simulink model "Battery_Model"  (R2019b)
settings: configuration reference "BMS_Sw_CodeGenConfig" (kept outside this file)
undefined symbols (not defined in the file): Battery, TempInit, ts
libraries: fl_lib x2765, nesl_utility x1565, ee_lib x384, simulink x384, BatteryPack_lib x3
(part 2 of 33)

== system Battery_Model/Battery_Pack/Battery_Pack_7Modules/Cell_3p1 ==
  BalCmd : Inport
  AmTmp : Inport  Port=2
  CellMonitoringUnit_1 : Subsystem
  CellMonitoringUnit_2 : Subsystem
  CellMonitoringUnit_3 : Subsystem
  Cell_Module_1 : Subsystem
  Cell_Module_2 : Subsystem
  Cell_Module_3 : Subsystem
  Data Type Conversion2 : DataTypeConversion  OutDataTypeStr=double
  Data Type Conversion3 : DataTypeConversion  OutDataTypeStr=single
  Data Type Conversion4 : DataTypeConversion  OutDataTypeStr=single
  Data Type Conversion5 : DataTypeConversion  OutDataTypeStr=single
  Vector Concatenate : Concatenate  NumInputs=3
  Vector Concatenate1 : Concatenate  NumInputs=3
  Cell+ : PMIOPort  Side=Right
  Cell- : PMIOPort  Port=2  Side=Right
  Cell_Voltages : Outport  VectorParamsAs1DForOutWhenUnconnected=off
  Cell_Temperatures : Outport  Port=2  VectorParamsAs1DForOutWhenUnconnected=off
  wires:
  Data Type Conversion4/1 -> [Module01_Volts]
  CellMonitoringUnit_1/1(CellVoltages) -> Data Type Conversion4/1
  Data Type Conversion2/1 -> CellMonitoringUnit_3/1(BalCmd), CellMonitoringUnit_2/1(BalCmd), CellMonitoringUnit_1/1(BalCmd)
  [Module01_Volts] -> Vector Concatenate/1  "Module01_Volts"
  Data Type Conversion5/1 -> [Module03_Volts]
  AmTmp/1 -> Cell_Module_3/1(AmbientTemp), Cell_Module_2/1(AmbientTemp), Cell_Module_1/1(AmbientTemp)
  CellMonitoringUnit_2/1(CellVoltages) -> Data Type Conversion3/1
  Data Type Conversion3/1 -> [Module02_Volts]
  Cell_Module_1/1(CellTemp) -> [Module01_Temps]
  Cell_Module_2/1(CellTemp) -> [Module02_Temps]
  BalCmd/1 -> Data Type Conversion2/1
  CellMonitoringUnit_3/1(CellVoltages) -> Data Type Conversion5/1
  [Module03_Volts] -> Vector Concatenate/3  "Module03_Volts"
  Vector Concatenate/1 -> Cell_Voltages/1
  [Module02_Volts] -> Vector Concatenate/2  "Module02_Volts"
  Cell_Module_3/1(CellTemp) -> [Module03_Temps]
  [Module03_Temps] -> Vector Concatenate1/3
  [Module01_Temps] -> Vector Concatenate1/1
  [Module02_Temps] -> Vector Concatenate1/2
  Vector Concatenate1/1 -> Cell_Temperatures/1
  connections:
  CellMonitoringUnit_1/LConn9 -- Cell_Module_1/RConn9
  Cell_Module_3/RConn6 -- CellMonitoringUnit_3/LConn6
  Cell_Module_2/RConn11 -- CellMonitoringUnit_2/LConn11
  Cell_Module_3/RConn9 -- CellMonitoringUnit_3/LConn9
  Cell_Module_2/RConn5 -- CellMonitoringUnit_2/LConn5
  CellMonitoringUnit_1/LConn13 -- Cell_Module_1/RConn13
  Cell_Module_2/RConn6 -- CellMonitoringUnit_2/LConn6
  Cell_Module_1/RConn17 -- Cell-/RConn1 -- CellMonitoringUnit_2/LConn17 -- CellMonitoringUnit_3/LConn17 -- Cell_Module_3/RConn17 -- Cell_Module_2/RConn17 -- CellMonitoringUnit_1/LConn17
  CellMonitoringUnit_1/LConn8 -- Cell_Module_1/RConn8
  Cell_Module_2/RConn13 -- CellMonitoringUnit_2/LConn13
  Cell_Module_2/RConn8 -- CellMonitoringUnit_2/LConn8
  CellMonitoringUnit_1/LConn1 -- Cell_Module_3/RConn1 -- CellMonitoringUnit_3/LConn1 -- Cell_Module_2/RConn1 -- CellMonitoringUnit_2/LConn1 -- Cell_Module_1/RConn1 -- Cell+/RConn1
  CellMonitoringUnit_1/LConn7 -- Cell_Module_1/RConn7
  Cell_Module_2/RConn10 -- CellMonitoringUnit_2/LConn10
  Cell_Module_3/RConn3 -- CellMonitoringUnit_3/LConn3
  Cell_Module_2/RConn14 -- CellMonitoringUnit_2/LConn14
  Cell_Module_2/RConn16 -- CellMonitoringUnit_2/LConn16
  Cell_Module_2/RConn12 -- CellMonitoringUnit_2/LConn12
  Cell_Module_2/RConn2 -- CellMonitoringUnit_2/LConn2
  Cell_Module_3/RConn4 -- CellMonitoringUnit_3/LConn4
  Cell_Module_3/RConn2 -- CellMonitoringUnit_3/LConn2
  Cell_Module_3/RConn8 -- CellMonitoringUnit_3/LConn8
  CellMonitoringUnit_1/LConn11 -- Cell_Module_1/RConn11
  Cell_Module_2/RConn9 -- CellMonitoringUnit_2/LConn9
  Cell_Module_3/RConn12 -- CellMonitoringUnit_3/LConn12
  CellMonitoringUnit_1/LConn3 -- Cell_Module_1/RConn3
  CellMonitoringUnit_1/LConn15 -- Cell_Module_1/RConn15
  Cell_Module_3/RConn7 -- CellMonitoringUnit_3/LConn7
  CellMonitoringUnit_1/LConn5 -- Cell_Module_1/RConn5
  Cell_Module_3/RConn15 -- CellMonitoringUnit_3/LConn15
  CellMonitoringUnit_1/LConn12 -- Cell_Module_1/RConn12
  CellMonitoringUnit_1/LConn10 -- Cell_Module_1/RConn10
  Cell_Module_2/RConn3 -- CellMonitoringUnit_2/LConn3
  CellMonitoringUnit_1/LConn6 -- Cell_Module_1/RConn6
  Cell_Module_2/RConn4 -- CellMonitoringUnit_2/LConn4
  Cell_Module_3/RConn10 -- CellMonitoringUnit_3/LConn10
  CellMonitoringUnit_1/LConn14 -- Cell_Module_1/RConn14
  CellMonitoringUnit_1/LConn4 -- Cell_Module_1/RConn4
  Cell_Module_3/RConn16 -- CellMonitoringUnit_3/LConn16
  Cell_Module_3/RConn11 -- CellMonitoringUnit_3/LConn11
  Cell_Module_3/RConn13 -- CellMonitoringUnit_3/LConn13
  Cell_Module_3/RConn14 -- CellMonitoringUnit_3/LConn14
  Cell_Module_3/RConn5 -- CellMonitoringUnit_3/LConn5
  Cell_Module_2/RConn15 -- CellMonitoringUnit_2/LConn15
  Cell_Module_2/RConn7 -- CellMonitoringUnit_2/LConn7
  CellMonitoringUnit_1/LConn2 -- Cell_Module_1/RConn2
  CellMonitoringUnit_1/LConn16 -- Cell_Module_1/RConn16

== system Battery_Model/Battery_Pack/Battery_Pack_1Module/Cell_3p/CellMonitoringUnit_1 ==
  BalCmd : Inport
  D{1..4,7..9,13..16} (11 alike) : fl_lib/Electrical/Electrical Elements/Diode  Vf=0.6 V  Ron=0.3 Ohm  Goff=1e-8 1/Ohm  i_specify=off  i_priority=High  i=0 A  i_nominal_specify=off  i_nominal_unit=A  i_nominal_value=1  v_specify=off  v_priority=None  v=0 V  v_nominal_specify=off  v_nominal_unit=V  v_nominal_value=1
      settings: LogSimulationData=on
  D{5..6,10..12} (5 alike) : fl_lib/Electrical/Electrical Elements/Diode  Vf=0.6 V  Ron=0.3 Ohm  Goff=1e-8 1/Ohm  i_specify=off  i_priority=None  i=0 A  i_nominal_specify=off  i_nominal_unit=A  i_nominal_value=1  v_specify=off  v_priority=None  v=0 V  v_nominal_specify=off  v_nominal_unit=V  v_nominal_value=1
      settings: LogSimulationData=on
  Data Type Conversion{,1..15} (16 alike) : DataTypeConversion  OutDataTypeStr=single
  PS-Simulink Converter{1..12,14..17} (16 alike) : nesl_utility/PS-Simulink Converter  PhysicalDomain=network_engine_domain  SubClassName=ps_output  LeftPortType=input  RightPortType=output  PseudoPeriodic=off  Frequencies=[]  Unit=V  AffineConversion=off
  R{1..16} (16 alike) : fl_lib/Electrical/Electrical Elements/Resistor  R=Battery.R_bleed Ohm  i_specify=off  i_priority=None  i=0 A  i_nominal_specify=off  i_nominal_unit=A  i_nominal_value=1  v_specify=off  v_priority=None  v=0 V  v_nominal_specify=off  v_nominal_unit=V  v_nominal_value=1
      R1 settings: LogSimulationData=on
  Selector : Selector  IndexOptions=Index vector (dialog)  Indices=1  OutputSizes=1
  Selector1 : Selector  IndexOptions=Index vector (dialog)  Indices=2  OutputSizes=1
  Selector10 : Selector  IndexOptions=Index vector (dialog)  Indices=6  OutputSizes=1
  Selector{3,8,11,15} (4 alike) : Selector  IndexOptions=Index vector (dialog)  Indices=4  OutputSizes=1
  Selector12 : Selector  IndexOptions=Index vector (dialog)  Indices=6  OutputSizes=1
  Selector13 : Selector  IndexOptions=Index vector (dialog)  Indices=2  OutputSizes=1
  Selector14 : Selector  IndexOptions=Index vector (dialog)  Indices=3  OutputSizes=1
  Selector2 : Selector  IndexOptions=Index vector (dialog)  Indices=3  OutputSizes=1
  Selector4 : Selector  IndexOptions=Index vector (dialog)  Indices=5  OutputSizes=1
  Selector5 : Selector  IndexOptions=Index vector (dialog)  Indices=6  OutputSizes=1
  Selector6 : Selector  IndexOptions=Index vector (dialog)  Indices=2  OutputSizes=1
  Selector7 : Selector  IndexOptions=Index vector (dialog)  Indices=3  OutputSizes=1
  Selector9 : Selector  IndexOptions=Index vector (dialog)  Indices=5  OutputSizes=1
  Simulink-PS Converter{1..12,14..17} (16 alike) : nesl_utility/Simulink-PS Converter  PhysicalDomain=network_engine_domain  SubClassName=ps_input  LeftPortType=input  RightPortType=output  PseudoPeriodic=off  Frequencies=[]  NoiseDistribution=none  NoiseParameters=[]  Unit=1  AffineConversion=off  FilteringAndDerivatives=zero  SimscapeFilterOrder=1  InputFilterTimeConstant=0.001  UdotUserProvided=1
  Switch{,1..15} (16 alike) : fl_lib/Electrical/Electrical Elements/Switch  R_closed=0.01 Ohm  G_open=1e-8 1/Ohm  Threshold=0  i_specify=off  i_priority=None  i=0 A  i_nominal_specify=off  i_nominal_unit=A  i_nominal_value=1  v_specify=off  v_priority=None  v=0 V  v_nominal_specify=off  v_nominal_unit=V  v_nominal_value=1
      settings: SourceProductName=Simscape
  Vector Concatenate : Concatenate  NumInputs=16
  Voltage Sensor{1..12,14..17} (16 alike) : fl_lib/Electrical/Electrical Sensors/Voltage Sensor
  Conn1 : PMIOPort  Side=Left
  Conn2 : PMIOPort  Port=2  Side=Left
  Conn3 : PMIOPort  Port=3  Side=Left
  Conn4 : PMIOPort  Port=4  Side=Left
  Conn5 : PMIOPort  Port=5  Side=Left
  Conn6 : PMIOPort  Port=6  Side=Left
  Conn7 : PMIOPort  Port=7  Side=Left
  Conn8 : PMIOPort  Port=8  Side=Left
  Conn9 : PMIOPort  Port=9  Side=Left
  Conn10 : PMIOPort  Port=10  Side=Left
  Conn11 : PMIOPort  Port=11  Side=Left
  Conn12 : PMIOPort  Port=12  Side=Left
  Conn13 : PMIOPort  Port=13  Side=Left
  Conn14 : PMIOPort  Port=14  Side=Left
  Conn15 : PMIOPort  Port=15  Side=Left
  Conn16 : PMIOPort  Port=16  Side=Left
  Conn17 : PMIOPort  Port=17  Side=Left
  CellVoltages : Outport  VectorParamsAs1DForOutWhenUnconnected=off
  wires:
  BalCmd/1 -> Selector/1, Selector1/1, Selector11/1, Selector15/1, Selector14/1, Selector13/1, Selector12/1, Selector10/1, Selector9/1, Selector8/1, Selector7/1, Selector6/1, Selector5/1, Selector4/1, Selector3/1, Selector2/1
  PS-Simulink Converter8/1 -> Data Type Conversion8/1  "Cell9_Volt"
  Selector5/1 -> Simulink-PS Converter6/1
  PS-Simulink Converter10/1 -> Data Type Conversion9/1  "Cell10_Volt"
  Selector9/1 -> Simulink-PS Converter10/1
  Data Type Conversion3/1 -> Vector Concatenate/4  "Cell4_Volt"
  Data Type Conversion12/1 -> Vector Concatenate/12  "Cell12_Volt"
  Selector6/1 -> Simulink-PS Converter7/1
  PS-Simulink Converter12/1 -> Data Type Conversion11/1  "Cell16_Volt"
  Data Type Conversion8/1 -> Vector Concatenate/9  "Cell9_Volt"
  Selector2/1 -> Simulink-PS Converter4/1
  Data Type Conversion/1 -> Vector Concatenate/1  "Cell1_Volt"
  Selector8/1 -> Simulink-PS Converter8/1
  Data Type Conversion15/1 -> Vector Concatenate/15  "Cell15_Volt"
  Data Type Conversion11/1 -> Vector Concatenate/16  "Cell16_Volt"
  Selector10/1 -> Simulink-PS Converter11/1
  PS-Simulink Converter15/1 -> Data Type Conversion14/1  "Cell14_Volt"
  Data Type Conversion4/1 -> Vector Concatenate/5  "Cell5_Volt"
  PS-Simulink Converter9/1 -> Data Type Conversion6/1  "Cell7_Volt"
  PS-Simulink Converter11/1 -> Data Type Conversion10/1  "Cell11_Volt"
  Data Type Conversion2/1 -> Vector Concatenate/3  "Cell3_Volt"
  Data Type Conversion7/1 -> Vector Concatenate/8  "Cell8_Volt"
  PS-Simulink Converter7/1 -> Data Type Conversion7/1  "Cell8_Volt"
  Selector7/1 -> Simulink-PS Converter9/1
  Selector12/1 -> Simulink-PS Converter14/1
  PS-Simulink Converter14/1 -> Data Type Conversion12/1  "Cell12_Volt"
  Selector15/1 -> Simulink-PS Converter16/1
  Selector14/1 -> Simulink-PS Converter17/1
  PS-Simulink Converter17/1 -> Data Type Conversion13/1  "Cell13_Volt"
  Data Type Conversion13/1 -> Vector Concatenate/13  "Cell13_Volt"
  PS-Simulink Converter16/1 -> Data Type Conversion15/1  "Cell15_Volt"
  Selector13/1 -> Simulink-PS Converter15/1
  Data Type Conversion1/1 -> Vector Concatenate/2  "Cell2_Volt"
  Data Type Conversion9/1 -> Vector Concatenate/10  "Cell10_Volt"
  PS-Simulink Converter6/1 -> Data Type Conversion5/1  "Cell6_Volt"
  PS-Simulink Converter4/1 -> Data Type Conversion1/1  "Cell2_Volt"
  Selector11/1 -> Simulink-PS Converter12/1
  Data Type Conversion14/1 -> Vector Concatenate/14  "Cell14_Volt"
  Vector Concatenate/1 -> CellVoltages/1
  Selector4/1 -> Simulink-PS Converter5/1
  Selector1/1 -> Simulink-PS Converter1/1
  PS-Simulink Converter2/1 -> Data Type Conversion/1  "Cell1_Volt"
  Selector3/1 -> Simulink-PS Converter2/1
  PS-Simulink Converter1/1 -> Data Type Conversion2/1  "Cell3_Volt"
  Selector/1 -> Simulink-PS Converter3/1
  PS-Simulink Converter3/1 -> Data Type Conversion3/1  "Cell4_Volt"
  PS-Simulink Converter5/1 -> Data Type Conversion4/1  "Cell5_Volt"
  Data Type Conversion5/1 -> Vector Concatenate/6  "Cell6_Volt"
  Data Type Conversion6/1 -> Vector Concatenate/7  "Cell7_Volt"
  Data Type Conversion10/1 -> Vector Concatenate/11  "Cell11_Volt"
  connections:
  Voltage Sensor10/RConn1 -- PS-Simulink Converter10/LConn1
  Simulink-PS Converter16/RConn1 -- Switch15/RConn1
  Switch15/RConn2 -- Voltage Sensor12/LConn1 -- Voltage Sensor17/RConn2 -- R16/LConn1 -- Conn16/RConn1
  R5/LConn1 -- Voltage Sensor5/LConn1 -- Voltage Sensor4/RConn2 -- Switch3/RConn2 -- Conn5/RConn1
  Switch12/RConn2 -- Voltage Sensor15/LConn1 -- Voltage Sensor14/RConn2 -- R13/LConn1 -- Conn13/RConn1
  Switch9/RConn2 -- R11/LConn1 -- Voltage Sensor11/LConn1 -- Voltage Sensor10/RConn2 -- Conn11/RConn1
  Switch7/LConn1 -- D8/RConn1
  Simulink-PS Converter10/RConn1 -- Switch9/RConn1
  Switch13/LConn1 -- D13/RConn1
  Voltage Sensor4/RConn1 -- PS-Simulink Converter3/LConn1
  Switch13/RConn2 -- R14/LConn1 -- Voltage Sensor16/LConn1 -- Voltage Sensor15/RConn2 -- Conn14/RConn1
  Voltage Sensor12/RConn1 -- PS-Simulink Converter12/LConn1
  Voltage Sensor14/LConn1 -- Voltage Sensor11/RConn2 -- R12/LConn1 -- Switch10/RConn2 -- Conn12/RConn1
  Simulink-PS Converter4/RConn1 -- Switch2/RConn1
  Simulink-PS Converter7/RConn1 -- Switch6/RConn1
  R11/RConn1 -- D11/LConn1
  Voltage Sensor14/RConn1 -- PS-Simulink Converter14/LConn1
  Voltage Sensor7/RConn1 -- PS-Simulink Converter9/LConn1
  Voltage Sensor9/RConn1 -- PS-Simulink Converter8/LConn1
  Switch9/LConn1 -- D10/RConn1
  R8/RConn1 -- D8/LConn1
  R9/RConn1 -- D9/LConn1
  Voltage Sensor16/RConn1 -- PS-Simulink Converter15/LConn1
  Simulink-PS Converter6/RConn1 -- Switch5/RConn1
  Simulink-PS Converter9/RConn1 -- Switch7/RConn1
  R7/RConn1 -- D7/LConn1
  Switch8/LConn1 -- D9/RConn1
  Simulink-PS Converter8/RConn1 -- Switch8/RConn1
  R3/RConn1 -- D3/LConn1
  Switch6/LConn1 -- D7/RConn1
  Switch4/RConn2 -- Voltage Sensor6/LConn1 -- Voltage Sensor5/RConn2 -- R6/LConn1 -- Conn6/RConn1
  Voltage Sensor17/RConn1 -- PS-Simulink Converter16/LConn1
  Switch3/LConn1 -- D4/RConn1
  Switch6/RConn2 -- R8/LConn1 -- Voltage Sensor7/RConn2 -- Voltage Sensor8/LConn1 -- Conn8/RConn1
  Switch/RConn2 -- R2/LConn1 -- Voltage Sensor2/LConn1 -- Voltage Sensor1/RConn2 -- Conn2/RConn1
  Switch15/LConn1 -- D15/RConn1
  Voltage Sensor9/RConn2 -- Voltage Sensor10/LConn1 -- R10/LConn1 -- Switch8/RConn2 -- Conn10/RConn1
  Voltage Sensor7/LConn1 -- Voltage Sensor6/RConn2 -- R7/LConn1 -- Switch5/RConn2 -- Conn7/RConn1
  Switch2/RConn2 -- R4/LConn1 -- Voltage Sensor4/LConn1 -- Voltage Sensor3/RConn2 -- Conn4/RConn1
  R12/RConn1 -- D12/LConn1
  Voltage Sensor11/RConn1 -- PS-Simulink Converter11/LConn1
  Simulink-PS Converter14/RConn1 -- Switch12/RConn1
  R14/RConn1 -- D14/LConn1
  Simulink-PS Converter17/RConn1 -- Switch14/RConn1
  Switch14/RConn2 -- R15/LConn1 -- Voltage Sensor17/LConn1 -- Voltage Sensor16/RConn2 -- Conn15/RConn1
  Switch12/LConn1 -- D12/RConn1
  Simulink-PS Converter2/RConn1 -- Switch3/RConn1
  R13/RConn1 -- D13/LConn1
  Switch14/LConn1 -- D14/RConn1
  Voltage Sensor15/RConn1 -- PS-Simulink Converter17/LConn1
  Switch11/RConn2 -- Voltage Sensor12/RConn2 -- Conn17/RConn1
  R15/RConn1 -- D15/LConn1
  Simulink-PS Converter15/RConn1 -- Switch13/RConn1
  Switch5/LConn1 -- D6/RConn1
  Switch7/RConn2 -- R9/LConn1 -- Voltage Sensor9/LConn1 -- Voltage Sensor8/RConn2 -- Conn9/RConn1
  Voltage Sensor8/RConn1 -- PS-Simulink Converter7/LConn1
  R1/LConn1 -- Voltage Sensor1/LConn1 -- Conn1/RConn1
  Voltage Sensor3/LConn1 -- Voltage Sensor2/RConn2 -- R3/LConn1 -- Switch1/RConn2 -- Conn3/RConn1
  Simulink-PS Converter12/RConn1 -- Switch11/RConn1
  Simulink-PS Converter1/RConn1 -- Switch1/RConn1
  PS-Simulink Converter2/LConn1 -- Voltage Sensor1/RConn1
  R4/RConn1 -- D4/LConn1
  Switch1/LConn1 -- D2/RConn1
  R2/RConn1 -- D2/LConn1
  Simulink-PS Converter5/RConn1 -- Switch4/RConn1
  Switch2/LConn1 -- D3/RConn1
  Simulink-PS Converter3/RConn1 -- Switch/RConn1
  Switch4/LConn1 -- D5/RConn1
  Voltage Sensor2/RConn1 -- PS-Simulink Converter4/LConn1
  R1/RConn1 -- D1/LConn1
  R5/RConn1 -- D5/LConn1
  Voltage Sensor3/RConn1 -- PS-Simulink Converter1/LConn1
  Switch/LConn1 -- D1/RConn1
  R6/RConn1 -- D6/LConn1
  Voltage Sensor5/RConn1 -- PS-Simulink Converter5/LConn1
  R10/RConn1 -- D10/LConn1
  Voltage Sensor6/RConn1 -- PS-Simulink Converter6/LConn1
  Simulink-PS Converter11/RConn1 -- Switch10/RConn1
  Switch10/LConn1 -- D11/RConn1
  R16/RConn1 -- D16/LConn1
  Switch11/LConn1 -- D16/RConn1

== system Battery_Model/Battery_Pack/Battery_Pack_1Module/Cell_3p/CellMonitoringUnit_2 ==
  BalCmd : Inport
  D{1..4,7..9,13..16} (11 alike) : fl_lib/Electrical/Electrical Elements/Diode  Vf=0.6 V  Ron=0.3 Ohm  Goff=1e-8 1/Ohm  i_specify=off  i_priority=High  i=0 A  i_nominal_specify=off  i_nominal_unit=A  i_nominal_value=1  v_specify=off  v_priority=None  v=0 V  v_nominal_specify=off  v_nominal_unit=V  v_nominal_value=1
      settings: LogSimulationData=on
  D{5..6,10..12} (5 alike) : fl_lib/Electrical/Electrical Elements/Diode  Vf=0.6 V  Ron=0.3 Ohm  Goff=1e-8 1/Ohm  i_specify=off  i_priority=None  i=0 A  i_nominal_specify=off  i_nominal_unit=A  i_nominal_value=1  v_specify=off  v_priority=None  v=0 V  v_nominal_specify=off  v_nominal_unit=V  v_nominal_value=1
      settings: LogSimulationData=on
  Data Type Conversion{,1..15} (16 alike) : DataTypeConversion  OutDataTypeStr=single
  PS-Simulink Converter{1..12,14..17} (16 alike) : nesl_utility/PS-Simulink Converter  PhysicalDomain=network_engine_domain  SubClassName=ps_output  LeftPortType=input  RightPortType=output  PseudoPeriodic=off  Frequencies=[]  Unit=V  AffineConversion=off
  R{1..16} (16 alike) : fl_lib/Electrical/Electrical Elements/Resistor  R=Battery.R_bleed Ohm  i_specify=off  i_priority=None  i=0 A  i_nominal_specify=off  i_nominal_unit=A  i_nominal_value=1  v_specify=off  v_priority=None  v=0 V  v_nominal_specify=off  v_nominal_unit=V  v_nominal_value=1
      R1 settings: LogSimulationData=on
  Selector : Selector  IndexOptions=Index vector (dialog)  Indices=1  OutputSizes=1
  Selector1 : Selector  IndexOptions=Index vector (dialog)  Indices=2  OutputSizes=1
  Selector10 : Selector  IndexOptions=Index vector (dialog)  Indices=6  OutputSizes=1
  Selector{3,8,11,15} (4 alike) : Selector  IndexOptions=Index vector (dialog)  Indices=4  OutputSizes=1
  Selector12 : Selector  IndexOptions=Index vector (dialog)  Indices=6  OutputSizes=1
  Selector13 : Selector  IndexOptions=Index vector (dialog)  Indices=2  OutputSizes=1
  Selector14 : Selector  IndexOptions=Index vector (dialog)  Indices=3  OutputSizes=1
  Selector2 : Selector  IndexOptions=Index vector (dialog)  Indices=3  OutputSizes=1
  Selector4 : Selector  IndexOptions=Index vector (dialog)  Indices=5  OutputSizes=1
  Selector5 : Selector  IndexOptions=Index vector (dialog)  Indices=6  OutputSizes=1
  Selector6 : Selector  IndexOptions=Index vector (dialog)  Indices=2  OutputSizes=1
  Selector7 : Selector  IndexOptions=Index vector (dialog)  Indices=3  OutputSizes=1
  Selector9 : Selector  IndexOptions=Index vector (dialog)  Indices=5  OutputSizes=1
  Simulink-PS Converter{1..12,14..17} (16 alike) : nesl_utility/Simulink-PS Converter  PhysicalDomain=network_engine_domain  SubClassName=ps_input  LeftPortType=input  RightPortType=output  PseudoPeriodic=off  Frequencies=[]  NoiseDistribution=none  NoiseParameters=[]  Unit=1  AffineConversion=off  FilteringAndDerivatives=zero  SimscapeFilterOrder=1  InputFilterTimeConstant=0.001  UdotUserProvided=1
  Switch{,1..15} (16 alike) : fl_lib/Electrical/Electrical Elements/Switch  R_closed=0.01 Ohm  G_open=1e-8 1/Ohm  Threshold=0  i_specify=off  i_priority=None  i=0 A  i_nominal_specify=off  i_nominal_unit=A  i_nominal_value=1  v_specify=off  v_priority=None  v=0 V  v_nominal_specify=off  v_nominal_unit=V  v_nominal_value=1
      settings: SourceProductName=Simscape
  Vector Concatenate : Concatenate  NumInputs=16
  Voltage Sensor{1..12,14..17} (16 alike) : fl_lib/Electrical/Electrical Sensors/Voltage Sensor
  Conn1 : PMIOPort  Side=Left
  Conn2 : PMIOPort  Port=2  Side=Left
  Conn3 : PMIOPort  Port=3  Side=Left
  Conn4 : PMIOPort  Port=4  Side=Left
  Conn5 : PMIOPort  Port=5  Side=Left
  Conn6 : PMIOPort  Port=6  Side=Left
  Conn7 : PMIOPort  Port=7  Side=Left
  Conn8 : PMIOPort  Port=8  Side=Left
  Conn9 : PMIOPort  Port=9  Side=Left
  Conn10 : PMIOPort  Port=10  Side=Left
  Conn11 : PMIOPort  Port=11  Side=Left
  Conn12 : PMIOPort  Port=12  Side=Left
  Conn13 : PMIOPort  Port=13  Side=Left
  Conn14 : PMIOPort  Port=14  Side=Left
  Conn15 : PMIOPort  Port=15  Side=Left
  Conn16 : PMIOPort  Port=16  Side=Left
  Conn17 : PMIOPort  Port=17  Side=Left
  CellVoltages : Outport  VectorParamsAs1DForOutWhenUnconnected=off
  wires:
  BalCmd/1 -> Selector/1, Selector1/1, Selector11/1, Selector15/1, Selector14/1, Selector13/1, Selector12/1, Selector10/1, Selector9/1, Selector8/1, Selector7/1, Selector6/1, Selector5/1, Selector4/1, Selector3/1, Selector2/1
  PS-Simulink Converter8/1 -> Data Type Conversion8/1  "Cell9_Volt"
  Selector5/1 -> Simulink-PS Converter6/1
  PS-Simulink Converter10/1 -> Data Type Conversion9/1  "Cell10_Volt"
  Selector9/1 -> Simulink-PS Converter10/1
  Data Type Conversion3/1 -> Vector Concatenate/4  "Cell4_Volt"
  Data Type Conversion12/1 -> Vector Concatenate/12  "Cell12_Volt"
  Selector6/1 -> Simulink-PS Converter7/1
  PS-Simulink Converter12/1 -> Data Type Conversion11/1  "Cell16_Volt"
  Data Type Conversion8/1 -> Vector Concatenate/9  "Cell9_Volt"
  Selector2/1 -> Simulink-PS Converter4/1
  Data Type Conversion/1 -> Vector Concatenate/1  "Cell1_Volt"
  Selector8/1 -> Simulink-PS Converter8/1
  Data Type Conversion15/1 -> Vector Concatenate/15  "Cell15_Volt"
  Data Type Conversion11/1 -> Vector Concatenate/16  "Cell16_Volt"
  Selector10/1 -> Simulink-PS Converter11/1
  PS-Simulink Converter15/1 -> Data Type Conversion14/1  "Cell14_Volt"
  Data Type Conversion4/1 -> Vector Concatenate/5  "Cell5_Volt"
  PS-Simulink Converter9/1 -> Data Type Conversion6/1  "Cell7_Volt"
  PS-Simulink Converter11/1 -> Data Type Conversion10/1  "Cell11_Volt"
  Data Type Conversion2/1 -> Vector Concatenate/3  "Cell3_Volt"
  Data Type Conversion7/1 -> Vector Concatenate/8  "Cell8_Volt"
  PS-Simulink Converter7/1 -> Data Type Conversion7/1  "Cell8_Volt"
  Selector7/1 -> Simulink-PS Converter9/1
  Selector12/1 -> Simulink-PS Converter14/1
  PS-Simulink Converter14/1 -> Data Type Conversion12/1  "Cell12_Volt"
  Selector15/1 -> Simulink-PS Converter16/1
  Selector14/1 -> Simulink-PS Converter17/1
  PS-Simulink Converter17/1 -> Data Type Conversion13/1  "Cell13_Volt"
  Data Type Conversion13/1 -> Vector Concatenate/13  "Cell13_Volt"
  PS-Simulink Converter16/1 -> Data Type Conversion15/1  "Cell15_Volt"
  Selector13/1 -> Simulink-PS Converter15/1
  Data Type Conversion1/1 -> Vector Concatenate/2  "Cell2_Volt"
  Data Type Conversion9/1 -> Vector Concatenate/10  "Cell10_Volt"
  PS-Simulink Converter6/1 -> Data Type Conversion5/1  "Cell6_Volt"
  PS-Simulink Converter4/1 -> Data Type Conversion1/1  "Cell2_Volt"
  Selector11/1 -> Simulink-PS Converter12/1
  Data Type Conversion14/1 -> Vector Concatenate/14  "Cell14_Volt"
  Vector Concatenate/1 -> CellVoltages/1
  Selector4/1 -> Simulink-PS Converter5/1
  Selector1/1 -> Simulink-PS Converter1/1
  PS-Simulink Converter2/1 -> Data Type Conversion/1  "Cell1_Volt"
  Selector3/1 -> Simulink-PS Converter2/1
  PS-Simulink Converter1/1 -> Data Type Conversion2/1  "Cell3_Volt"
  Selector/1 -> Simulink-PS Converter3/1
  PS-Simulink Converter3/1 -> Data Type Conversion3/1  "Cell4_Volt"
  PS-Simulink Converter5/1 -> Data Type Conversion4/1  "Cell5_Volt"
  Data Type Conversion5/1 -> Vector Concatenate/6  "Cell6_Volt"
  Data Type Conversion6/1 -> Vector Concatenate/7  "Cell7_Volt"
  Data Type Conversion10/1 -> Vector Concatenate/11  "Cell11_Volt"
  connections:
  Voltage Sensor10/RConn1 -- PS-Simulink Converter10/LConn1
  Simulink-PS Converter16/RConn1 -- Switch15/RConn1
  Switch15/RConn2 -- Voltage Sensor12/LConn1 -- Voltage Sensor17/RConn2 -- R16/LConn1 -- Conn16/RConn1
  R5/LConn1 -- Voltage Sensor5/LConn1 -- Voltage Sensor4/RConn2 -- Switch3/RConn2 -- Conn5/RConn1
  Switch12/RConn2 -- Voltage Sensor15/LConn1 -- Voltage Sensor14/RConn2 -- R13/LConn1 -- Conn13/RConn1
  Switch9/RConn2 -- R11/LConn1 -- Voltage Sensor11/LConn1 -- Voltage Sensor10/RConn2 -- Conn11/RConn1
  Switch7/LConn1 -- D8/RConn1
  Simulink-PS Converter10/RConn1 -- Switch9/RConn1
  Switch13/LConn1 -- D13/RConn1
  Voltage Sensor4/RConn1 -- PS-Simulink Converter3/LConn1
  Switch13/RConn2 -- R14/LConn1 -- Voltage Sensor16/LConn1 -- Voltage Sensor15/RConn2 -- Conn14/RConn1
  Voltage Sensor12/RConn1 -- PS-Simulink Converter12/LConn1
  Voltage Sensor14/LConn1 -- Voltage Sensor11/RConn2 -- R12/LConn1 -- Switch10/RConn2 -- Conn12/RConn1
  Simulink-PS Converter4/RConn1 -- Switch2/RConn1
  Simulink-PS Converter7/RConn1 -- Switch6/RConn1
  R11/RConn1 -- D11/LConn1
  Voltage Sensor14/RConn1 -- PS-Simulink Converter14/LConn1
  Voltage Sensor7/RConn1 -- PS-Simulink Converter9/LConn1
  Voltage Sensor9/RConn1 -- PS-Simulink Converter8/LConn1
  Switch9/LConn1 -- D10/RConn1
  R8/RConn1 -- D8/LConn1
  R9/RConn1 -- D9/LConn1
  Voltage Sensor16/RConn1 -- PS-Simulink Converter15/LConn1
  Simulink-PS Converter6/RConn1 -- Switch5/RConn1
  Simulink-PS Converter9/RConn1 -- Switch7/RConn1
  R7/RConn1 -- D7/LConn1
  Switch8/LConn1 -- D9/RConn1
  Simulink-PS Converter8/RConn1 -- Switch8/RConn1
  R3/RConn1 -- D3/LConn1
  Switch6/LConn1 -- D7/RConn1
  Switch4/RConn2 -- Voltage Sensor6/LConn1 -- Voltage Sensor5/RConn2 -- R6/LConn1 -- Conn6/RConn1
  Voltage Sensor17/RConn1 -- PS-Simulink Converter16/LConn1
  Switch3/LConn1 -- D4/RConn1
  Switch6/RConn2 -- R8/LConn1 -- Voltage Sensor7/RConn2 -- Voltage Sensor8/LConn1 -- Conn8/RConn1
  Switch/RConn2 -- R2/LConn1 -- Voltage Sensor2/LConn1 -- Voltage Sensor1/RConn2 -- Conn2/RConn1
  Switch15/LConn1 -- D15/RConn1
  Voltage Sensor9/RConn2 -- Voltage Sensor10/LConn1 -- R10/LConn1 -- Switch8/RConn2 -- Conn10/RConn1
  Voltage Sensor7/LConn1 -- Voltage Sensor6/RConn2 -- R7/LConn1 -- Switch5/RConn2 -- Conn7/RConn1
  Switch2/RConn2 -- R4/LConn1 -- Voltage Sensor4/LConn1 -- Voltage Sensor3/RConn2 -- Conn4/RConn1
  R12/RConn1 -- D12/LConn1
  Voltage Sensor11/RConn1 -- PS-Simulink Converter11/LConn1
  Simulink-PS Converter14/RConn1 -- Switch12/RConn1
  R14/RConn1 -- D14/LConn1
  Simulink-PS Converter17/RConn1 -- Switch14/RConn1
  Switch14/RConn2 -- R15/LConn1 -- Voltage Sensor17/LConn1 -- Voltage Sensor16/RConn2 -- Conn15/RConn1
  Switch12/LConn1 -- D12/RConn1
  Simulink-PS Converter2/RConn1 -- Switch3/RConn1
  R13/RConn1 -- D13/LConn1
  Switch14/LConn1 -- D14/RConn1
  Voltage Sensor15/RConn1 -- PS-Simulink Converter17/LConn1
  Switch11/RConn2 -- Voltage Sensor12/RConn2 -- Conn17/RConn1
  R15/RConn1 -- D15/LConn1
  Simulink-PS Converter15/RConn1 -- Switch13/RConn1
  Switch5/LConn1 -- D6/RConn1
  Switch7/RConn2 -- R9/LConn1 -- Voltage Sensor9/LConn1 -- Voltage Sensor8/RConn2 -- Conn9/RConn1
  Voltage Sensor8/RConn1 -- PS-Simulink Converter7/LConn1
  R1/LConn1 -- Voltage Sensor1/LConn1 -- Conn1/RConn1
  Voltage Sensor3/LConn1 -- Voltage Sensor2/RConn2 -- R3/LConn1 -- Switch1/RConn2 -- Conn3/RConn1
  Simulink-PS Converter12/RConn1 -- Switch11/RConn1
  Simulink-PS Converter1/RConn1 -- Switch1/RConn1
  PS-Simulink Converter2/LConn1 -- Voltage Sensor1/RConn1
  R4/RConn1 -- D4/LConn1
  Switch1/LConn1 -- D2/RConn1
  R2/RConn1 -- D2/LConn1
  Simulink-PS Converter5/RConn1 -- Switch4/RConn1
  Switch2/LConn1 -- D3/RConn1
  Simulink-PS Converter3/RConn1 -- Switch/RConn1
  Switch4/LConn1 -- D5/RConn1
  Voltage Sensor2/RConn1 -- PS-Simulink Converter4/LConn1
  R1/RConn1 -- D1/LConn1
  R5/RConn1 -- D5/LConn1
  Voltage Sensor3/RConn1 -- PS-Simulink Converter1/LConn1
  Switch/LConn1 -- D1/RConn1
  R6/RConn1 -- D6/LConn1
  Voltage Sensor5/RConn1 -- PS-Simulink Converter5/LConn1
  R10/RConn1 -- D10/LConn1
  Voltage Sensor6/RConn1 -- PS-Simulink Converter6/LConn1
  Simulink-PS Converter11/RConn1 -- Switch10/RConn1
  Switch10/LConn1 -- D11/RConn1
  R16/RConn1 -- D16/LConn1
  Switch11/LConn1 -- D16/RConn1

== system Battery_Model/Battery_Pack/Battery_Pack_1Module/Cell_3p/CellMonitoringUnit_3 ==
  BalCmd : Inport
  D{1..4,7..9,13..16} (11 alike) : fl_lib/Electrical/Electrical Elements/Diode  Vf=0.6 V  Ron=0.3 Ohm  Goff=1e-8 1/Ohm  i_specify=off  i_priority=High  i=0 A  i_nominal_specify=off  i_nominal_unit=A  i_nominal_value=1  v_specify=off  v_priority=None  v=0 V  v_nominal_specify=off  v_nominal_unit=V  v_nominal_value=1
      settings: LogSimulationData=on
  D{5..6,10..12} (5 alike) : fl_lib/Electrical/Electrical Elements/Diode  Vf=0.6 V  Ron=0.3 Ohm  Goff=1e-8 1/Ohm  i_specify=off  i_priority=None  i=0 A  i_nominal_specify=off  i_nominal_unit=A  i_nominal_value=1  v_specify=off  v_priority=None  v=0 V  v_nominal_specify=off  v_nominal_unit=V  v_nominal_value=1
      settings: LogSimulationData=on
  Data Type Conversion{,1..15} (16 alike) : DataTypeConversion  OutDataTypeStr=single
  PS-Simulink Converter{1..12,14..17} (16 alike) : nesl_utility/PS-Simulink Converter  PhysicalDomain=network_engine_domain  SubClassName=ps_output  LeftPortType=input  RightPortType=output  PseudoPeriodic=off  Frequencies=[]  Unit=V  AffineConversion=off
  R{1..16} (16 alike) : fl_lib/Electrical/Electrical Elements/Resistor  R=Battery.R_bleed Ohm  i_specify=off  i_priority=None  i=0 A  i_nominal_specify=off  i_nominal_unit=A  i_nominal_value=1  v_specify=off  v_priority=None  v=0 V  v_nominal_specify=off  v_nominal_unit=V  v_nominal_value=1
      R1 settings: LogSimulationData=on
  Selector : Selector  IndexOptions=Index vector (dialog)  Indices=1  OutputSizes=1
  Selector1 : Selector  IndexOptions=Index vector (dialog)  Indices=2  OutputSizes=1
  Selector10 : Selector  IndexOptions=Index vector (dialog)  Indices=6  OutputSizes=1
  Selector{3,8,11,15} (4 alike) : Selector  IndexOptions=Index vector (dialog)  Indices=4  OutputSizes=1
  Selector12 : Selector  IndexOptions=Index vector (dialog)  Indices=6  OutputSizes=1
  Selector13 : Selector  IndexOptions=Index vector (dialog)  Indices=2  OutputSizes=1
  Selector14 : Selector  IndexOptions=Index vector (dialog)  Indices=3  OutputSizes=1
  Selector2 : Selector  IndexOptions=Index vector (dialog)  Indices=3  OutputSizes=1
  Selector4 : Selector  IndexOptions=Index vector (dialog)  Indices=5  OutputSizes=1
  Selector5 : Selector  IndexOptions=Index vector (dialog)  Indices=6  OutputSizes=1
  Selector6 : Selector  IndexOptions=Index vector (dialog)  Indices=2  OutputSizes=1
  Selector7 : Selector  IndexOptions=Index vector (dialog)  Indices=3  OutputSizes=1
  Selector9 : Selector  IndexOptions=Index vector (dialog)  Indices=5  OutputSizes=1
  Simulink-PS Converter{1..12,14..17} (16 alike) : nesl_utility/Simulink-PS Converter  PhysicalDomain=network_engine_domain  SubClassName=ps_input  LeftPortType=input  RightPortType=output  PseudoPeriodic=off  Frequencies=[]  NoiseDistribution=none  NoiseParameters=[]  Unit=1  AffineConversion=off  FilteringAndDerivatives=zero  SimscapeFilterOrder=1  InputFilterTimeConstant=0.001  UdotUserProvided=1
  Switch{,1..15} (16 alike) : fl_lib/Electrical/Electrical Elements/Switch  R_closed=0.01 Ohm  G_open=1e-8 1/Ohm  Threshold=0  i_specify=off  i_priority=None  i=0 A  i_nominal_specify=off  i_nominal_unit=A  i_nominal_value=1  v_specify=off  v_priority=None  v=0 V  v_nominal_specify=off  v_nominal_unit=V  v_nominal_value=1
      settings: SourceProductName=Simscape
  Vector Concatenate : Concatenate  NumInputs=16
  Voltage Sensor{1..12,14..17} (16 alike) : fl_lib/Electrical/Electrical Sensors/Voltage Sensor
  Conn1 : PMIOPort  Side=Left
  Conn2 : PMIOPort  Port=2  Side=Left
  Conn3 : PMIOPort  Port=3  Side=Left
  Conn4 : PMIOPort  Port=4  Side=Left
  Conn5 : PMIOPort  Port=5  Side=Left
  Conn6 : PMIOPort  Port=6  Side=Left
  Conn7 : PMIOPort  Port=7  Side=Left
  Conn8 : PMIOPort  Port=8  Side=Left
  Conn9 : PMIOPort  Port=9  Side=Left
  Conn10 : PMIOPort  Port=10  Side=Left
  Conn11 : PMIOPort  Port=11  Side=Left
  Conn12 : PMIOPort  Port=12  Side=Left
  Conn13 : PMIOPort  Port=13  Side=Left
  Conn14 : PMIOPort  Port=14  Side=Left
  Conn15 : PMIOPort  Port=15  Side=Left
  Conn16 : PMIOPort  Port=16  Side=Left
  Conn17 : PMIOPort  Port=17  Side=Left
  CellVoltages : Outport  VectorParamsAs1DForOutWhenUnconnected=off
  wires:
  BalCmd/1 -> Selector/1, Selector1/1, Selector11/1, Selector15/1, Selector14/1, Selector13/1, Selector12/1, Selector10/1, Selector9/1, Selector8/1, Selector7/1, Selector6/1, Selector5/1, Selector4/1, Selector3/1, Selector2/1
  PS-Simulink Converter8/1 -> Data Type Conversion8/1  "Cell9_Volt"
  Selector5/1 -> Simulink-PS Converter6/1
  PS-Simulink Converter10/1 -> Data Type Conversion9/1  "Cell10_Volt"
  Selector9/1 -> Simulink-PS Converter10/1
  Data Type Conversion3/1 -> Vector Concatenate/4  "Cell4_Volt"
  Data Type Conversion12/1 -> Vector Concatenate/12  "Cell12_Volt"
  Selector6/1 -> Simulink-PS Converter7/1
  PS-Simulink Converter12/1 -> Data Type Conversion11/1  "Cell16_Volt"
  Data Type Conversion8/1 -> Vector Concatenate/9  "Cell9_Volt"
  Selector2/1 -> Simulink-PS Converter4/1
  Data Type Conversion/1 -> Vector Concatenate/1  "Cell1_Volt"
  Selector8/1 -> Simulink-PS Converter8/1
  Data Type Conversion15/1 -> Vector Concatenate/15  "Cell15_Volt"
  Data Type Conversion11/1 -> Vector Concatenate/16  "Cell16_Volt"
  Selector10/1 -> Simulink-PS Converter11/1
  PS-Simulink Converter15/1 -> Data Type Conversion14/1  "Cell14_Volt"
  Data Type Conversion4/1 -> Vector Concatenate/5  "Cell5_Volt"
  PS-Simulink Converter9/1 -> Data Type Conversion6/1  "Cell7_Volt"
  PS-Simulink Converter11/1 -> Data Type Conversion10/1  "Cell11_Volt"
  Data Type Conversion2/1 -> Vector Concatenate/3  "Cell3_Volt"
  Data Type Conversion7/1 -> Vector Concatenate/8  "Cell8_Volt"
  PS-Simulink Converter7/1 -> Data Type Conversion7/1  "Cell8_Volt"
  Selector7/1 -> Simulink-PS Converter9/1
  Selector12/1 -> Simulink-PS Converter14/1
  PS-Simulink Converter14/1 -> Data Type Conversion12/1  "Cell12_Volt"
  Selector15/1 -> Simulink-PS Converter16/1
  Selector14/1 -> Simulink-PS Converter17/1
  PS-Simulink Converter17/1 -> Data Type Conversion13/1  "Cell13_Volt"
  Data Type Conversion13/1 -> Vector Concatenate/13  "Cell13_Volt"
  PS-Simulink Converter16/1 -> Data Type Conversion15/1  "Cell15_Volt"
  Selector13/1 -> Simulink-PS Converter15/1
  Data Type Conversion1/1 -> Vector Concatenate/2  "Cell2_Volt"
  Data Type Conversion9/1 -> Vector Concatenate/10  "Cell10_Volt"
  PS-Simulink Converter6/1 -> Data Type Conversion5/1  "Cell6_Volt"
  PS-Simulink Converter4/1 -> Data Type Conversion1/1  "Cell2_Volt"
  Selector11/1 -> Simulink-PS Converter12/1
  Data Type Conversion14/1 -> Vector Concatenate/14  "Cell14_Volt"
  Vector Concatenate/1 -> CellVoltages/1
  Selector4/1 -> Simulink-PS Converter5/1
  Selector1/1 -> Simulink-PS Converter1/1
  PS-Simulink Converter2/1 -> Data Type Conversion/1  "Cell1_Volt"
  Selector3/1 -> Simulink-PS Converter2/1
  PS-Simulink Converter1/1 -> Data Type Conversion2/1  "Cell3_Volt"
  Selector/1 -> Simulink-PS Converter3/1
  PS-Simulink Converter3/1 -> Data Type Conversion3/1  "Cell4_Volt"
  PS-Simulink Converter5/1 -> Data Type Conversion4/1  "Cell5_Volt"
  Data Type Conversion5/1 -> Vector Concatenate/6  "Cell6_Volt"
  Data Type Conversion6/1 -> Vector Concatenate/7  "Cell7_Volt"
  Data Type Conversion10/1 -> Vector Concatenate/11  "Cell11_Volt"
  connections:
  Voltage Sensor10/RConn1 -- PS-Simulink Converter10/LConn1
  Simulink-PS Converter16/RConn1 -- Switch15/RConn1
  Switch15/RConn2 -- Voltage Sensor12/LConn1 -- Voltage Sensor17/RConn2 -- R16/LConn1 -- Conn16/RConn1
  R5/LConn1 -- Voltage Sensor5/LConn1 -- Voltage Sensor4/RConn2 -- Switch3/RConn2 -- Conn5/RConn1
  Switch12/RConn2 -- Voltage Sensor15/LConn1 -- Voltage Sensor14/RConn2 -- R13/LConn1 -- Conn13/RConn1
  Switch9/RConn2 -- R11/LConn1 -- Voltage Sensor11/LConn1 -- Voltage Sensor10/RConn2 -- Conn11/RConn1
  Switch7/LConn1 -- D8/RConn1
  Simulink-PS Converter10/RConn1 -- Switch9/RConn1
  Switch13/LConn1 -- D13/RConn1
  Voltage Sensor4/RConn1 -- PS-Simulink Converter3/LConn1
  Switch13/RConn2 -- R14/LConn1 -- Voltage Sensor16/LConn1 -- Voltage Sensor15/RConn2 -- Conn14/RConn1
  Voltage Sensor12/RConn1 -- PS-Simulink Converter12/LConn1
  Voltage Sensor14/LConn1 -- Voltage Sensor11/RConn2 -- R12/LConn1 -- Switch10/RConn2 -- Conn12/RConn1
  Simulink-PS Converter4/RConn1 -- Switch2/RConn1
  Simulink-PS Converter7/RConn1 -- Switch6/RConn1
  R11/RConn1 -- D11/LConn1
  Voltage Sensor14/RConn1 -- PS-Simulink Converter14/LConn1
  Voltage Sensor7/RConn1 -- PS-Simulink Converter9/LConn1
  Voltage Sensor9/RConn1 -- PS-Simulink Converter8/LConn1
  Switch9/LConn1 -- D10/RConn1
  R8/RConn1 -- D8/LConn1
  R9/RConn1 -- D9/LConn1
  Voltage Sensor16/RConn1 -- PS-Simulink Converter15/LConn1
  Simulink-PS Converter6/RConn1 -- Switch5/RConn1
  Simulink-PS Converter9/RConn1 -- Switch7/RConn1
  R7/RConn1 -- D7/LConn1
  Switch8/LConn1 -- D9/RConn1
  Simulink-PS Converter8/RConn1 -- Switch8/RConn1
  R3/RConn1 -- D3/LConn1
  Switch6/LConn1 -- D7/RConn1
  Switch4/RConn2 -- Voltage Sensor6/LConn1 -- Voltage Sensor5/RConn2 -- R6/LConn1 -- Conn6/RConn1
  Voltage Sensor17/RConn1 -- PS-Simulink Converter16/LConn1
  Switch3/LConn1 -- D4/RConn1
  Switch6/RConn2 -- R8/LConn1 -- Voltage Sensor7/RConn2 -- Voltage Sensor8/LConn1 -- Conn8/RConn1
  Switch/RConn2 -- R2/LConn1 -- Voltage Sensor2/LConn1 -- Voltage Sensor1/RConn2 -- Conn2/RConn1
  Switch15/LConn1 -- D15/RConn1
  Voltage Sensor9/RConn2 -- Voltage Sensor10/LConn1 -- R10/LConn1 -- Switch8/RConn2 -- Conn10/RConn1
  Voltage Sensor7/LConn1 -- Voltage Sensor6/RConn2 -- R7/LConn1 -- Switch5/RConn2 -- Conn7/RConn1
  Switch2/RConn2 -- R4/LConn1 -- Voltage Sensor4/LConn1 -- Voltage Sensor3/RConn2 -- Conn4/RConn1
  R12/RConn1 -- D12/LConn1
  Voltage Sensor11/RConn1 -- PS-Simulink Converter11/LConn1
  Simulink-PS Converter14/RConn1 -- Switch12/RConn1
  R14/RConn1 -- D14/LConn1
  Simulink-PS Converter17/RConn1 -- Switch14/RConn1
  Switch14/RConn2 -- R15/LConn1 -- Voltage Sensor17/LConn1 -- Voltage Sensor16/RConn2 -- Conn15/RConn1
  Switch12/LConn1 -- D12/RConn1
  Simulink-PS Converter2/RConn1 -- Switch3/RConn1
  R13/RConn1 -- D13/LConn1
  Switch14/LConn1 -- D14/RConn1
  Voltage Sensor15/RConn1 -- PS-Simulink Converter17/LConn1
  Switch11/RConn2 -- Voltage Sensor12/RConn2 -- Conn17/RConn1
  R15/RConn1 -- D15/LConn1
  Simulink-PS Converter15/RConn1 -- Switch13/RConn1
  Switch5/LConn1 -- D6/RConn1
  Switch7/RConn2 -- R9/LConn1 -- Voltage Sensor9/LConn1 -- Voltage Sensor8/RConn2 -- Conn9/RConn1
  Voltage Sensor8/RConn1 -- PS-Simulink Converter7/LConn1
  R1/LConn1 -- Voltage Sensor1/LConn1 -- Conn1/RConn1
  Voltage Sensor3/LConn1 -- Voltage Sensor2/RConn2 -- R3/LConn1 -- Switch1/RConn2 -- Conn3/RConn1
  Simulink-PS Converter12/RConn1 -- Switch11/RConn1
  Simulink-PS Converter1/RConn1 -- Switch1/RConn1
  PS-Simulink Converter2/LConn1 -- Voltage Sensor1/RConn1
  R4/RConn1 -- D4/LConn1
  Switch1/LConn1 -- D2/RConn1
  R2/RConn1 -- D2/LConn1
  Simulink-PS Converter5/RConn1 -- Switch4/RConn1
  Switch2/LConn1 -- D3/RConn1
  Simulink-PS Converter3/RConn1 -- Switch/RConn1
  Switch4/LConn1 -- D5/RConn1
  Voltage Sensor2/RConn1 -- PS-Simulink Converter4/LConn1
  R1/RConn1 -- D1/LConn1
  R5/RConn1 -- D5/LConn1
  Voltage Sensor3/RConn1 -- PS-Simulink Converter1/LConn1
  Switch/LConn1 -- D1/RConn1
  R6/RConn1 -- D6/LConn1
  Voltage Sensor5/RConn1 -- PS-Simulink Converter5/LConn1
  R10/RConn1 -- D10/LConn1
  Voltage Sensor6/RConn1 -- PS-Simulink Converter6/LConn1
  Simulink-PS Converter11/RConn1 -- Switch10/RConn1
  Switch10/LConn1 -- D11/RConn1
  R16/RConn1 -- D16/LConn1
  Switch11/LConn1 -- D16/RConn1
